simulink model "tarefa_6_3"  (R2023b)
settings: Solver=VariableStepAuto  StartTime=0.0  StopTime=1  FixedStep=passo  RelTol=1e-3
InitFcn:
  | %% Parametros da rede
  | Vabc = 380;
  | Vrede = Vabc*sqrt(2/3);
  | Frede = 60;
  | Vdc = 700;
  | fsw = 6e3;
  | 
  | %% Parametros PLL
  | Winit = 2*pi*60;
  | wn_srf = 2*pi*60/3;
  | epsilon = 1/sqrt(2);
  | 
  | Ki_pll = (wn_srf^2)/Vrede;
  | Kp_pll = 2*epsilon*sqrt(Ki_pll/Vrede);
  | 
  | %% Parametros Filtro
  | Lg = 406.3e-6;
  | Cf = 31.1744e-6;
  | Rd = 1;
  | Lf = Lg;
  | L = Lg+Lf;
  | R = 2*pi*Frede*L/40;
  | 
  | %% Malha Interna PI
  | fcd = fsw/20;
  | Kp_int_pi = 2*pi*fcd*L;
  | kp = 2*pi*fcd*L-R;
  | Ki_int = 2*pi*fcd*R;
  | wnL = 2*pi*Frede*L;
undefined symbols (not defined in the file): plecs
settings Model: Creator=unknow  LastModifiedBy=unknow

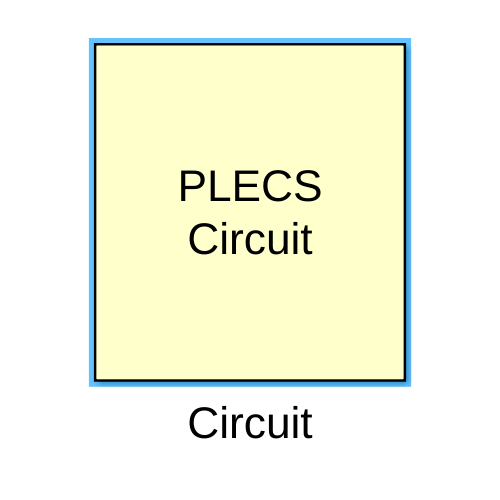
[thumbnail: Simulink's stored preview of the top-level diagram]
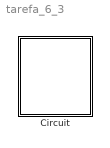
== system tarefa_6_3 ==
  Circuit : Subsystem  LoadFcn=plecs('sl', 200);  InitFcn=plecs('sl', 214);  StartFcn=plecs('sl', 208);  StopFcn=plecs('sl', 209);  mask(PlecsCircuit){PLECSData=<binary blob, 14040 chars, not shown>}
      mask prompts: PLECSData "PLECS Data (Do not delete or modify!)"
      mask init:
      | % PLACE CUSTOM INITIALIZATIONS ABOVE
      | % DO NOT REMOVE
      | plecs('sl', 215);
      | % DO NOT REMOVE
      settings: CopyFcn=plecs('sl', 203);  DeleteFcn=plecs('sl', 205);  UndoDeleteFcn=plecs('sl', 206);  PreSaveFcn=plecs('sl', 211);  PostSaveFcn=plecs('sl', 201);  NameChangeFcn=plecs('sl', 210);  DestroyFcn=plecs('sl', 207);  PreCopyFcn=plecs('sl', 216);  OpenFcn=plecs('sl', 202);  ErrorFcn=plerrorfcn
      mask Help: eval('plecs(''help'', ''qthelp:///creatingacircuit.html'')')
      mask Display: disp('PLECS\nCircuit')

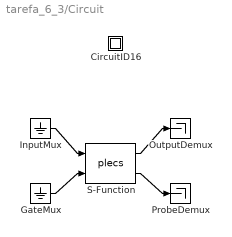
== system tarefa_6_3/Circuit ==
  " CircuitID16 " : Subsystem
  " GateMux " : Ground
  " InputMux " : Ground
  " OutputDemux " : Terminator
  " ProbeDemux " : Terminator
  " S-Function " : S-Function  FunctionName=plecs  SFunctionDeploymentMode=off  EnableBusSupport=off
  wires:
  " InputMux "/1 -> " S-Function "/1
  " GateMux "/1 -> " S-Function "/2
  " S-Function "/1 -> " OutputDemux "/1
  " S-Function "/2 -> " ProbeDemux "/1

== system tarefa_6_3/Circuit/ CircuitID16  ==
